simulink model "disturbanceEffectOn_first_order_open"  (R2023b)
settings: Solver=VariableStepAuto  StartTime=0.0  StopTime=10.0  RelTol=1e-3
settings Model: Creator=reemb  LastModifiedBy=reemb

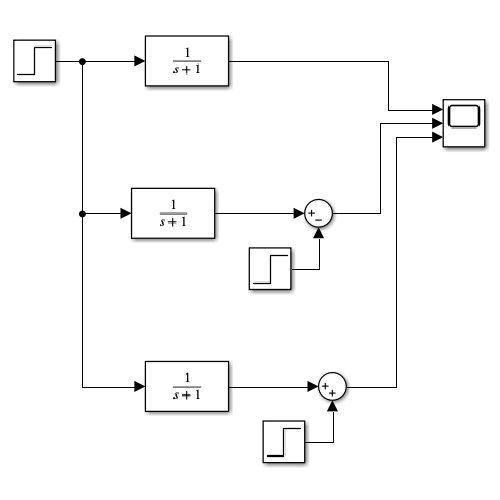
[thumbnail: Simulink's stored preview of the top-level diagram]
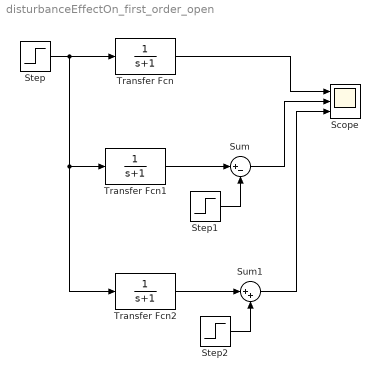
== system disturbanceEffectOn_first_order_open ==
  Scope : Scope  NumInputPorts=3
  Step : Step  SampleTime=0
  Step1 : Step  Time=3  SampleTime=0
  Step2 : Step  Time=3  SampleTime=0
  Sum : Sum  Inputs=|+-
  Sum1 : Sum  Inputs=|++
  Transfer Fcn : TransferFcn  Denominator=[1 1]
  Transfer Fcn1 : TransferFcn  Denominator=[1 1]
  Transfer Fcn2 : TransferFcn  Denominator=[1 1]
  wires:
  Transfer Fcn/1 -> Scope/1
  Transfer Fcn1/1 -> Sum/1
  Step1/1 -> Sum/2
  Sum/1 -> Scope/2
  Sum1/1 -> Scope/3
  Step2/1 -> Sum1/2
  Transfer Fcn2/1 -> Sum1/1
  Step/1 -> Transfer Fcn/1, Transfer Fcn2/1, Transfer Fcn1/1
